simulink model "BP2"  (Simulink 8.5)
settings: Solver=FixedStepDiscrete  SolverMode=SingleTasking  StartTime=0.0  StopTime=6e-3  FixedStep=Ts  MaxStep=3.90625e-06  RelTol=1e-3  AbsTol=1e-3
values from neighbouring files (symbols this model uses):
  alfa = (711-1)/711    (= 0.998593530239)    [BP2IP3.m]    (also in BP2param.m)
  Amax = 2    [BP2IP3.m]    (also in BP2param.m)
  Ampl = 0.5-pi/256    (= 0.487728153697)    [BP2IP3.m]    (also in BP2param.m)
  b = 0.125    [BP2IP3.m]    (also in BP2param.m)
  b2 = 0.125    [BP2IP3.m]    (also in BP2param.m)
  b3 = 0.25    [BP2IP3.m]    (also in BP2param.m)
  delta = 0.1e-9    (= 1e-10)    [BP2IP3.m]    (also in BP2param.m)
  finrad = Fin*2*pi    (= 67246496.3813)    [BP2param.m]
  GBW = 250e6    (= 250000000)    [BP2IP3.m]    (also in BP2param.m)
  k = 1.38e-23    [BP2IP3.m]    (also in BP2param.m)
  sr = 280e6    (= 280000000)    [BP2IP3.m]    (also in BP2param.m)
  Temp = 300    [BP2IP3.m]    (also in BP2param.m)
  Ts = 1/Fs    (= 2.33644859813e-08)    [BP2IP3.m]    (also in BP2param.m)
  Vref = 1    [BP2IP3.m]    (also in BP2param.m)
undefined symbols (not defined in the file or in its folder): slew
undefined symbols (not defined in the file): Cf, clock, noise1
CloseFcn:
  | ;slview('closediagram',bdroot);
settings Model: Creator=thaodang  LastModifiedBy=thaodang
settings DataIOCC: LimitDataPoints=off  SaveOutput=off  SaveTime=off
settings OptimizationCC: BlockReduction=off  BooleanDataType=off  ExpressionDepthLimit=128
settings DebuggingCC: SaveWithParameterizedLinksMsg=none  SignalResolutionControl=TryResolveAllWithWarning  MultiTaskDSMMsg=warning  MultiTaskCondExecSysMsg=none  FcnCallInpInsideContextMsg=EnableAllAsError  StateNameClashWarn=none  StrictBusMsg=None
settings HardwareCC: TargetUnknown=on
settings RTWCC: TemplateMakefile=grt.tmf

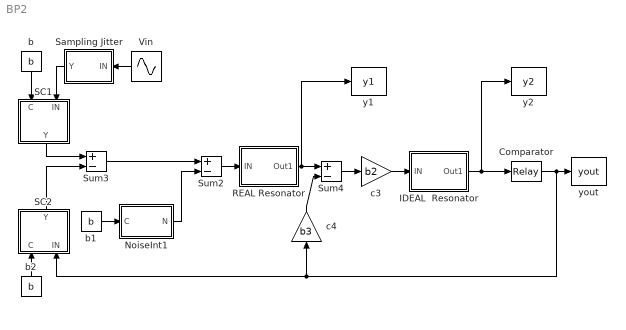
== system BP2 ==
  Comparator : Relay  OnOutputValue=Vref  OffOutputValue=-Vref
  IDEAL  Resonator : Subsystem  mask(Integrator){Ts=Ts}
      mask prompts: Ts "Sample Time:"
      mask help: Ideal discrete resonator with delay.
      mask Help:
      | Parameters:
      | Ts:       Sample time
      mask Display: dpoly([0 0 -1], [1 0 1], 'z-')
  NoiseInt1 : Subsystem  mask(OpAmp Noise){seed=sum(clock)^1/111, Ts=Ts, noise=noise1}
      mask prompts: seed "Random Number Seed:"; Ts "Sample Time:"; noise "Op-amp Noise Std. Dev.:"
      mask Display: disp('OpNoise')
  REAL Resonator : Subsystem  mask(Integrator){Ts=Ts, alfa=alfa, Amax=Amax, sr=sr, GBW=GBW}
      mask prompts: Ts "Sample Time:"; alfa "Finite Gain:"; Amax "Saturation:"; sr "Slew Rate:"; GBW "Gain-Bandwidth"
      mask help:
      | Real discrete integrator with delay.
      | Models op-amp saturation and slew rate.
      mask Help:
      | Parameters:
      | Ts:       Sample time
      | G:         Finite op-amp gain (ideal op-amp G=1)
      | Amax:  Saturation value
      | sr:       slew rate in V/s
      mask Display: dpoly([0 0 -1], [1 0 1], 'z-')
  SC1 : Subsystem  mask(kT/C Noise){Ts=Ts, Ci=Cf, Temp=Temp, k=k, seed=sum(clock)}
      mask prompts: Ts "Sample Time:"; Ci "Integrating Capacitance:"; Temp "Absolute Temperature:"; k "Boltzman Constant:"; seed "Random Number Seed:"
      mask help:
      | Models the kT/Cs noise of a switched capacitance Cs.
      | IN input: the input signal line
      | C input:   accepts the coefficient WITH SIGN (Cs/Ci)
      mask Help:
      | Block parameters:
      | Ts:        Sample time
      | Ci:        Integrating Capacitance
      | Temp:   Absolute Temperature in Kelvin
      | k:         Boltzmann Constant
      | seed:    Initial seed for random number generator
      | Outputs the noisy signal.
      mask Display: disp('kT/C')
  SC2 : Subsystem  mask(kT/C Noise){Ts=Ts, Ci=Cf, Temp=Temp, k=k, seed=2.11*sum(clock)}
      mask prompts: Ts "Sample Time:"; Ci "Integrating Capacitance:"; Temp "Absolute Temperature:"; k "Boltzman Constant:"; seed "Random Number Seed:"
      mask help:
      | Models the kT/Cs noise of a switched capacitance Cs.
      | IN input: the input signal line
      | C input:   accepts the coefficient WITH SIGN (Cs/Ci)
      mask Help:
      | Block parameters:
      | Ts:        Sample time
      | Ci:        Integrating Capacitance
      | Temp:   Absolute Temperature in Kelvin
      | k:         Boltzmann Constant
      | seed:    Initial seed for random number generator
      | Outputs the noisy signal.
      mask Display: disp('kT/C')
  Sampling Jitter : Subsystem  mask(Jitter){Ts=Ts, delta=delta, seed=(sum(clock))^3.33}
      mask prompts: Ts "Sample Time:"; delta "Sampling Jitter:"; seed "Random Number Seed:"
      mask help:
      | Models the kT/Cs noise of a switched capacitance Cs.
      | IN input: the input signal line
      | C input:   accepts the coefficient WITH SIGN (Cs/Ci)
      mask Help:
      | Block parameters:
      | Ts:        Sample time
      | Ci:        Integrating Capacitance
      | Temp:   Absolute Temperature in Kelvin
      | k:         Boltzmann Constant
      | seed:    Initial seed for random number generator
      | Outputs the noisy signal.
      mask Display: disp('Jitter')
  Sum2 : Sum  Inputs=+-  SaturateOnIntegerOverflow=on  InputSameDT=on  OutDataTypeStr=Inherit: Same as first input
  Sum3 : Sum  Inputs=+-  SaturateOnIntegerOverflow=on  InputSameDT=on  OutDataTypeStr=Inherit: Same as first input
  Sum4 : Sum  Inputs=+-  SaturateOnIntegerOverflow=on  InputSameDT=on  OutDataTypeStr=Inherit: Same as first input
  Vin : Sin  Amplitude=Ampl  Frequency=finrad  SampleTime=0
  b : Constant  Value=b
  b1 : Constant  Value=b
  b2 : Constant  Value=b
  c3 : Gain  Gain=b2  SaturateOnIntegerOverflow=on  OutDataTypeStr=Inherit: Same as input  ParamDataTypeStr=Inherit: Same as input
  c4 : Gain  Gain=b3  SaturateOnIntegerOverflow=on  OutDataTypeStr=Inherit: Same as input  ParamDataTypeStr=Inherit: Same as input
  y1 : ToWorkspace  VariableName=y1  SampleTime=-1
  y2 : ToWorkspace  VariableName=y2  SampleTime=-1
  yout : ToWorkspace  VariableName=yout  SampleTime=-1
  wires:
  Sum2/1 -> REAL Resonator/1(IN)
  Sum4/1 -> c3/1
  c3/1 -> IDEAL  Resonator/1(IN)
  NoiseInt1/1(N) -> Sum2/2
  b1/1 -> NoiseInt1/1(C)
  Sum3/1 -> Sum2/1
  SC1/1(Y) -> Sum3/1
  b/1 -> SC1/1(C)
  SC2/1(Y) -> Sum3/2
  Sampling Jitter/1(Y) -> SC1/2(IN)
  Vin/1 -> Sampling Jitter/1(IN)
  b2/1 -> SC2/1(C)
  REAL Resonator/1(Out1) -> Sum4/1, y1/1
  Comparator/1 -> yout/1, SC2/2(IN), c4/1
  IDEAL  Resonator/1(Out1) -> Comparator/1, y2/1
  c4/1 -> Sum4/2

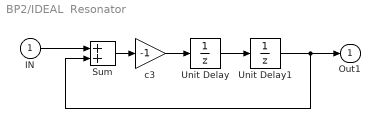
== system BP2/IDEAL  Resonator ==
  IN : Inport
  Sum : Sum  SaturateOnIntegerOverflow=on  InputSameDT=on  OutDataTypeStr=Inherit: Same as first input
  Unit Delay : UnitDelay  SampleTime=Ts
  Unit Delay1 : UnitDelay  SampleTime=Ts
  c3 : Gain  Gain=-1  SaturateOnIntegerOverflow=on  OutDataTypeStr=Inherit: Same as input  ParamDataTypeStr=Inherit: Same as input
  Out1 : Outport
  wires:
  IN/1 -> Sum/1
  Unit Delay/1 -> Unit Delay1/1
  Unit Delay1/1 -> Out1/1, Sum/2
  Sum/1 -> c3/1
  c3/1 -> Unit Delay/1

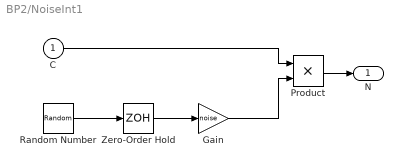
== system BP2/NoiseInt1 ==
  C : Inport
  Gain : Gain  Gain=noise  SaturateOnIntegerOverflow=on  OutDataTypeStr=Inherit: Same as input  ParamDataTypeStr=Inherit: Same as input
  Product : Product  SaturateOnIntegerOverflow=on  RndMeth=Zero  InputSameDT=on  OutDataTypeStr=Inherit: Same as first input
  Random Number : RandomNumber  Seed=seed  SampleTime=Ts
  Zero-Order Hold : ZeroOrderHold  SampleTime=Ts
  N : Outport  InitialOutput=0
  wires:
  Random Number/1 -> Zero-Order Hold/1
  Zero-Order Hold/1 -> Gain/1
  Product/1 -> N/1
  Gain/1 -> Product/2
  C/1 -> Product/1

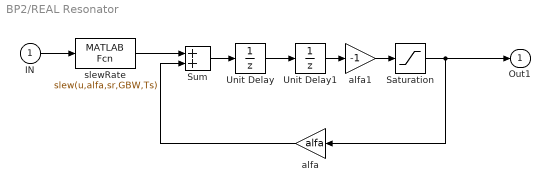
== system BP2/REAL Resonator ==
  IN : Inport
  Saturation : Saturate  UpperLimit=Amax  LowerLimit=-Amax
  Sum : Sum  SaturateOnIntegerOverflow=on  InputSameDT=on  OutDataTypeStr=Inherit: Same as first input
  Unit Delay : UnitDelay  SampleTime=Ts
  Unit Delay1 : UnitDelay  SampleTime=Ts
  alfa : Gain  Gain=alfa  SaturateOnIntegerOverflow=on  OutDataTypeStr=Inherit: Same as input  ParamDataTypeStr=Inherit: Same as input
  alfa1 : Gain  Gain=-1  SaturateOnIntegerOverflow=on  OutDataTypeStr=Inherit: Same as input  ParamDataTypeStr=Inherit: Same as input
  slewRate : MATLABFcn  MATLABFcn=slew(u,alfa,sr,GBW,Ts)
  Out1 : Outport
  wires:
  Sum/1 -> Unit Delay/1
  Saturation/1 -> Out1/1, alfa/1
  IN/1 -> slewRate/1
  slewRate/1 -> Sum/1
  alfa/1 -> Sum/2
  Unit Delay/1 -> Unit Delay1/1
  Unit Delay1/1 -> alfa1/1
  alfa1/1 -> Saturation/1

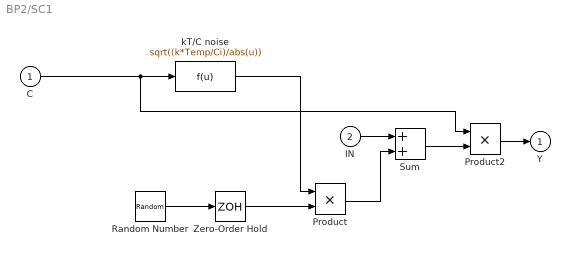
== system BP2/SC1 ==
  C : Inport
  IN : Inport  Port=2
  Product : Product  SaturateOnIntegerOverflow=on  RndMeth=Zero  InputSameDT=on  OutDataTypeStr=Inherit: Same as first input
  Product2 : Product  SaturateOnIntegerOverflow=on  RndMeth=Zero  InputSameDT=on  OutDataTypeStr=Inherit: Same as first input
  Random Number : RandomNumber  Seed=seed  SampleTime=Ts
  Sum : Sum  SaturateOnIntegerOverflow=on  InputSameDT=on  OutDataTypeStr=Inherit: Same as first input
  Zero-Order Hold : ZeroOrderHold  SampleTime=Ts
  kT/C noise : Fcn  Expr=sqrt((k*Temp/Ci)/abs(u))
  Y : Outport  InitialOutput=0
  wires:
  Random Number/1 -> Zero-Order Hold/1
  C/1 -> Product2/1, kT/C noise/1
  Zero-Order Hold/1 -> Product/2
  kT/C noise/1 -> Product/1
  Sum/1 -> Product2/2
  IN/1 -> Sum/1
  Product2/1 -> Y/1
  Product/1 -> Sum/2

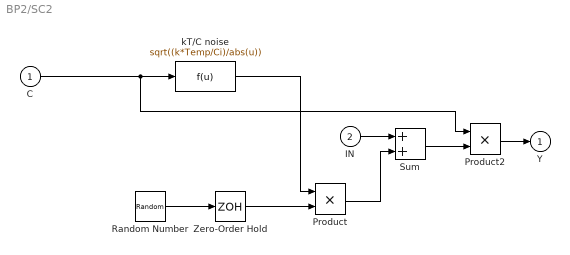
== system BP2/SC2 ==
  C : Inport
  IN : Inport  Port=2
  Product : Product  SaturateOnIntegerOverflow=on  RndMeth=Zero  InputSameDT=on  OutDataTypeStr=Inherit: Same as first input
  Product2 : Product  SaturateOnIntegerOverflow=on  RndMeth=Zero  InputSameDT=on  OutDataTypeStr=Inherit: Same as first input
  Random Number : RandomNumber  Seed=seed  SampleTime=Ts
  Sum : Sum  SaturateOnIntegerOverflow=on  InputSameDT=on  OutDataTypeStr=Inherit: Same as first input
  Zero-Order Hold : ZeroOrderHold  SampleTime=Ts
  kT/C noise : Fcn  Expr=sqrt((k*Temp/Ci)/abs(u))
  Y : Outport  InitialOutput=0
  wires:
  Random Number/1 -> Zero-Order Hold/1
  C/1 -> Product2/1, kT/C noise/1
  Zero-Order Hold/1 -> Product/2
  kT/C noise/1 -> Product/1
  Sum/1 -> Product2/2
  IN/1 -> Sum/1
  Product2/1 -> Y/1
  Product/1 -> Sum/2

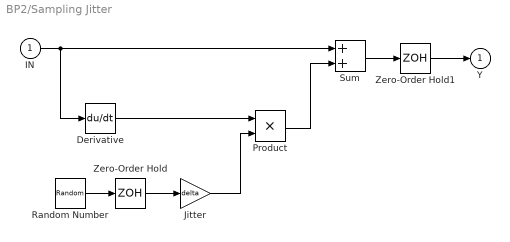
== system BP2/Sampling Jitter ==
  IN : Inport
  Derivative : Derivative
  Jitter : Gain  Gain=delta  SaturateOnIntegerOverflow=on  OutDataTypeStr=Inherit: Same as input  ParamDataTypeStr=Inherit: Same as input
  Product : Product  SaturateOnIntegerOverflow=on  RndMeth=Zero  InputSameDT=on  OutDataTypeStr=Inherit: Same as first input
  Random Number : RandomNumber  Seed=seed  SampleTime=Ts
  Sum : Sum  SaturateOnIntegerOverflow=on  InputSameDT=on  OutDataTypeStr=Inherit: Same as first input
  Zero-Order Hold : ZeroOrderHold  SampleTime=Ts
  Zero-Order Hold1 : ZeroOrderHold  SampleTime=Ts
  Y : Outport  InitialOutput=0
  wires:
  IN/1 -> Sum/1, Derivative/1
  Random Number/1 -> Zero-Order Hold/1
  Derivative/1 -> Product/1
  Zero-Order Hold/1 -> Jitter/1
  Jitter/1 -> Product/2
  Product/1 -> Sum/2
  Sum/1 -> Zero-Order Hold1/1
  Zero-Order Hold1/1 -> Y/1
